simulink model "s360159_sim_MPC"  (R2025b)
settings: Solver=VariableStepAuto  StartTime=0.0  StopTime=t_sim  RelTol=1e-3
values from neighbouring files (symbols this model uses):
  C = [1 0]    [s360159_MPC.mat]    (also in s360159_design.m = minreal(zpk(tf(S,R,Ts))))
  md =     [s360159_MPC.mat]
  Ts = 0.005    [s360159.mat]    (also in s360159_MPC.mat = 0.05; s360159_design.m)
libraries: cstblocks x1
settings Model: Creator=giovannimasi  LastModifiedBy=giovannimasi

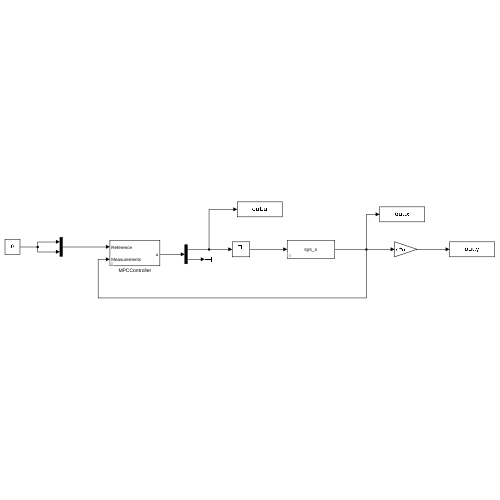
[thumbnail: Simulink's stored preview of the top-level diagram]
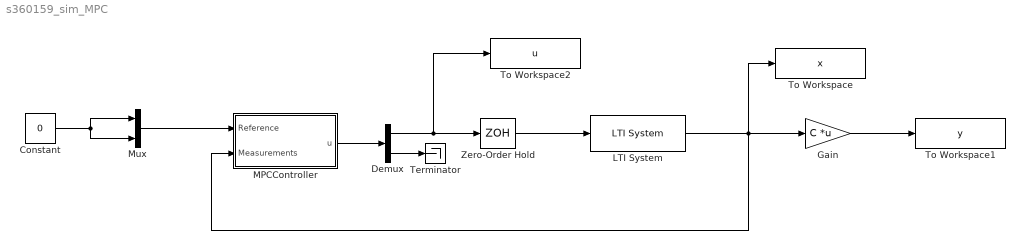
== system s360159_sim_MPC ==
  Constant : Constant  Value=0
  Demux : Demux  Outputs=2
  Gain : Gain  Gain=C  Multiplication=Matrix(K*u)
  LTI System : cstblocks/LTI System  sys=sys_x  IC=x0  PadeOrder=0
  MPCController : Subsystem  mask{md=md}
      mask prompts: md "MPCData"
  Mux : Mux  Inputs=2
  Terminator : Terminator
  To Workspace : ToWorkspace  VariableName=x  SaveFormat=Timeseries  SampleTime=Ts
  To Workspace1 : ToWorkspace  VariableName=y  SaveFormat=Timeseries  SampleTime=Ts
  To Workspace2 : ToWorkspace  VariableName=u  SaveFormat=Timeseries  SampleTime=Ts
  Zero-Order Hold : ZeroOrderHold  SampleTime=Ts
  wires:
  Mux/1 -> MPCController/1(Reference)
  Constant/1 -> Mux/1, Mux/2
  MPCController/1(u) -> Demux/1
  Demux/2 -> Terminator/1
  Demux/1 -> To Workspace2/1, Zero-Order Hold/1
  Zero-Order Hold/1 -> LTI System/1
  LTI System/1 -> To Workspace/1, MPCController/2(Measurements), Gain/1
  Gain/1 -> To Workspace1/1

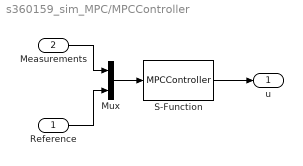
== system s360159_sim_MPC/MPCController ==
  Reference : Inport
  Measurements : Inport  Port=2
  Mux : Mux  Inputs=2
  S-Function : S-Function  FunctionName=MPCController  Parameters=md  SFunctionDeploymentMode=off  EnableBusSupport=off
  u : Outport
  wires:
  Mux/1 -> S-Function/1
  Measurements/1 -> Mux/1
  Reference/1 -> Mux/2
  S-Function/1 -> u/1
